simulink model "Q8_Simulation"  (R2022b)
settings: Solver=VariableStepAuto  StartTime=0.0  StopTime=25  RelTol=1e-3
undefined symbols (not defined in the file): A, B, C, K, P
settings Model: Creator=amirz  LastModifiedBy=amirz

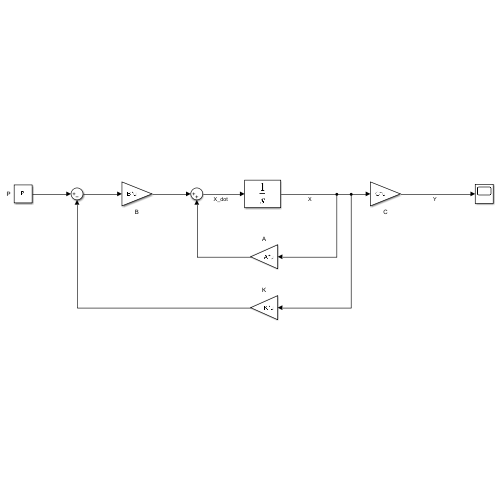
[thumbnail: Simulink's stored preview of the top-level diagram]
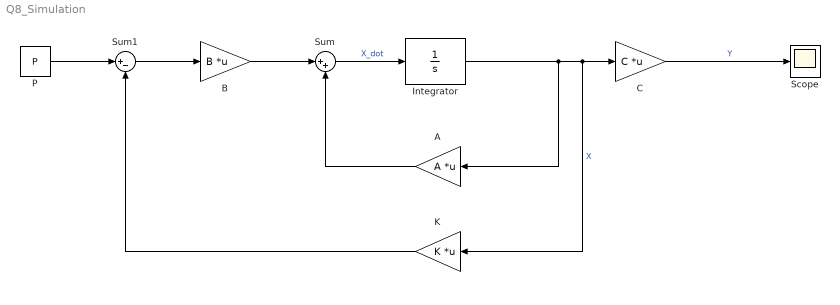
== system Q8_Simulation ==
  A : Gain  Gain=A  Multiplication=Matrix(K*u)
  B : Gain  Gain=B  Multiplication=Matrix(K*u)
  C : Gain  Gain=C  Multiplication=Matrix(K*u)
  Integrator : Integrator
  K : Gain  Gain=K  Multiplication=Matrix(K*u)
  P : Constant  Value=P
  Scope : Scope
  Sum : Sum  Inputs=|++
  Sum1 : Sum  Inputs=|+-
  wires:
  Integrator/1 -> A/1, K/1, C/1  "X"
  B/1 -> Sum/1
  K/1 -> Sum1/2
  Sum1/1 -> B/1
  A/1 -> Sum/2
  C/1 -> Scope/1  "Y"
  Sum/1 -> Integrator/1  "X_dot"
  P/1 -> Sum1/1
